simulink model "Session3_PID_OS_simulink"  (R2014a)
settings: Solver=ode45  StartTime=0.0  StopTime=20  RelTol=1e-3
settings Model: Creator=Omar Emad  LastModifiedBy=Omar Emad

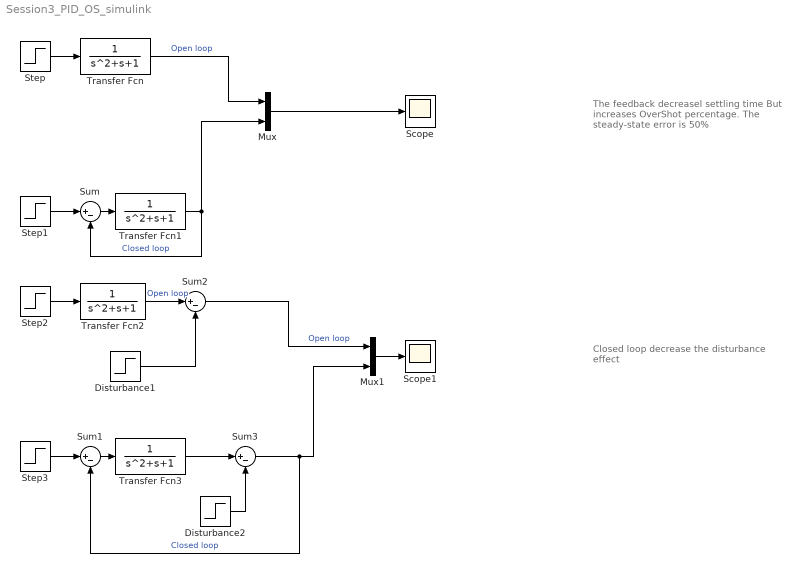
== system Session3_PID_OS_simulink ==
  note: The feedback decreasel settling time
      | But increases OverShot percentage.
      | The steady-state error is 50%
  note: Closed loop decrease the disturbance
      | effect
  Disturbance1 : Step  Time=4  After=0.2  SampleTime=0
  Disturbance2 : Step  Time=4  After=0.2  SampleTime=0
  Mux : Mux  Inputs=2
  Mux1 : Mux  Inputs=2
  Scope : Scope
  Scope1 : Scope
  Step{,1..3} (4 alike) : Step  SampleTime=0
  Sum{,1..3} (4 alike) : Sum  Inputs=|+-
  Transfer Fcn{,1..3} (4 alike) : TransferFcn  Denominator=[1 1 1]
  wires:
  Step/1 -> Transfer Fcn/1
  Transfer Fcn1/1 -> Sum/2, Mux/2  "Closed loop"
  Step1/1 -> Sum/1
  Sum/1 -> Transfer Fcn1/1
  Mux/1 -> Scope/1
  Transfer Fcn/1 -> Mux/1  "Open loop"
  Step2/1 -> Transfer Fcn2/1
  Transfer Fcn3/1 -> Sum3/1
  Step3/1 -> Sum1/1
  Sum1/1 -> Transfer Fcn3/1
  Mux1/1 -> Scope1/1
  Transfer Fcn2/1 -> Sum2/1  "Open loop"
  Sum2/1 -> Mux1/1  "Open loop"
  Disturbance1/1 -> Sum2/2
  Disturbance2/1 -> Sum3/2
  Sum3/1 -> Sum1/2, Mux1/2  "Closed loop"
